simulink model "block06"  (R2019a)
settings: Solver=VariableStepAuto  StartTime=0.0  StopTime=10.0  RelTol=1e-3
libraries: block05 x2
settings Model: Creator=b1991  LastModifiedBy=b1991
settings DataIOCC: InspectSignalLogs=on

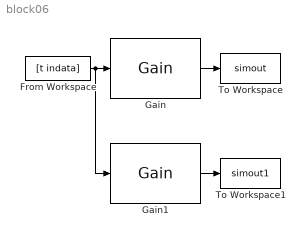
== system block06 ==
  From Workspace : FromWorkspace  VariableName=[t indata]  OutDataTypeStr=double  SampleTime=0
  Gain : block05/Gain  mask{G1=3}
      link override Gain: Gain=G1
  Gain1 : block05/Gain  mask{G1=6}
      link override Gain: Gain=G1
  To Workspace : ToWorkspace  VariableName=simout  SaveFormat=Timeseries  SampleTime=-1
  To Workspace1 : ToWorkspace  VariableName=simout1  SaveFormat=Timeseries  SampleTime=-1
  wires:
  From Workspace/1 -> Gain1/1, Gain/1
  Gain/1 -> To Workspace/1
  Gain1/1 -> To Workspace1/1
